simulink model "Regen_Model"  (R2023b)
settings: Solver=VariableStepAuto  StartTime=0.0  StopTime=10.0  RelTol=1e-3
undefined symbols (not defined in the file): DiscIntNeverNeededParam
settings Model: Creator=bglen  LastModifiedBy=bglen

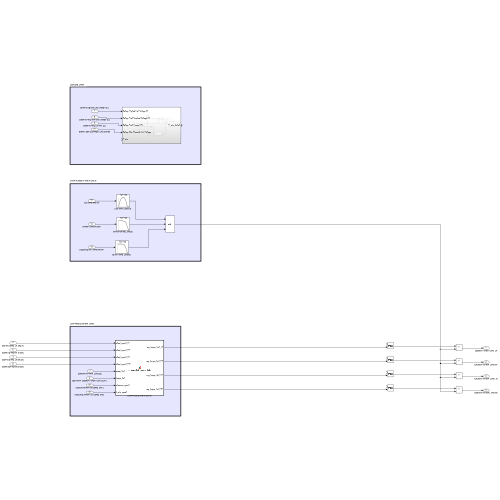
[thumbnail: Simulink's stored preview of the top-level diagram]
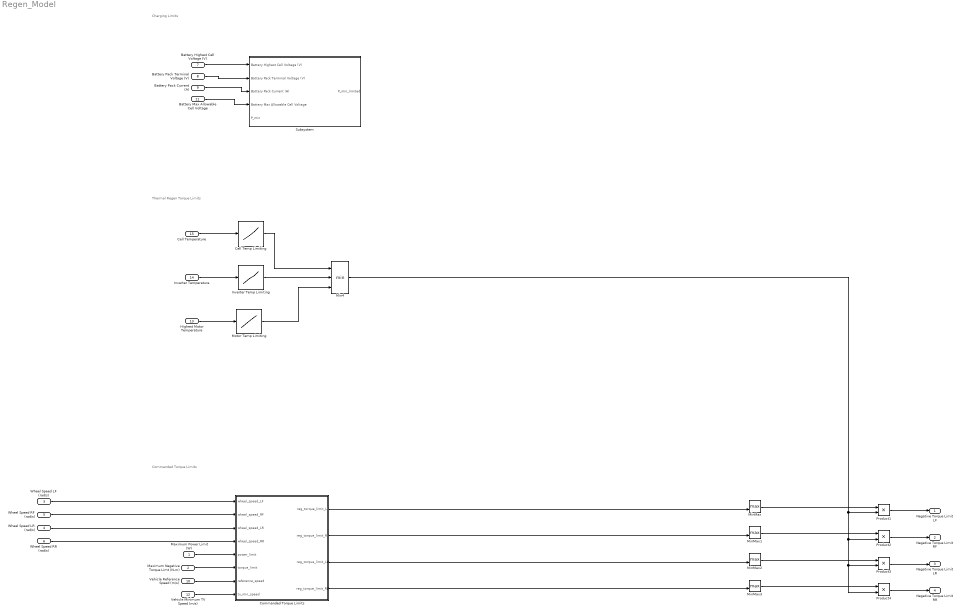
== system Regen_Model ==
  note: Commanded Torque Limits
  note: Thermal Regen Torque Limits
  note: Charging Limits
  Maximum Power Limit (W) : Inport
  Maximum Negative Torque Limt (N-m) : Inport  Port=2
  Wheel Speed LF (rad/s) : Inport  Port=3
  Wheel Speed LR (rad/s) : Inport  Port=4
  Wheel Speed RF (rad/s) : Inport  Port=5
  Wheel Speed RR (rad/s) : Inport  Port=6
  Battery Highest Cell Voltage (V) : Inport  Port=7
  Battery Pack Terminal Voltage (V) : Inport  Port=8
  Battery Pack Current (A) : Inport  Port=9
  Vehicle Reference Speed (m/s) : Inport  Port=10
  Battery Max Allowable Cell Voltage : Inport  Port=11
  Vehicle Minimum TV Speed (m/s) : Inport  Port=12
  Highest Motor Temperature : Inport  Port=13
  Inverter Temperature : Inport  Port=14
  Cell Temperature : Inport  Port=15
  Cell Temp Limiting : Lookup_n-D  NumberOfTableDimensions=1  BreakpointsForDimension1=[-15;-10;-5;0;5;10;15;20;25;30;35;40;45;50;55;60]  BreakpointsForDimension1Spacing=10  Table=[0;0.3;0.6;0.75;0.9;1;1;1;1;0.9;0.8;0.5;0.2;0.05;0;0]  InternalRulePriority=Speed  RndMeth=Simplest
  Commanded Torque Limits : MATLAB Function  TreatAsAtomicUnit=on
  Inverter Temp Limiting : Lookup_n-D  NumberOfTableDimensions=1  BreakpointsForDimension1=[0;10;20;30;40;50;60;70;80;90;100;110;120;130]  BreakpointsForDimension1Spacing=10  Table=[1;1;1;1;1;1;0.98;0.95;0.9;0.8;0.6;0.3;0.1;0]  InternalRulePriority=Speed  RndMeth=Simplest
  Min4 : MinMax  Inputs=3
  MinMax{,1..3} (4 alike) : MinMax  Function=max  Inputs=2
  Motor Temp Limiting : Lookup_n-D  NumberOfTableDimensions=1  BreakpointsForDimension1=[0;10;20;30;40;50;60;70;80;90;100;110;120;130;140]  BreakpointsForDimension1Spacing=10  Table=[1;1;1;1;1;1;1;0.98;0.95;0.9;0.8;0.6;0.3;0.1;0]  InternalRulePriority=Speed  RndMeth=Simplest
  Product{1..4} (4 alike) : Product
  Subsystem : Subsystem
  Negative Torque Limit LF : Outport
  Negative Torque Limit RF : Outport  Port=2
  Negative Torque Limit LR : Outport  Port=3
  Negative Torque Limit RR : Outport  Port=4
  wires:
  Product1/1 -> Negative Torque Limit LF/1
  Product2/1 -> Negative Torque Limit RF/1
  Product3/1 -> Negative Torque Limit LR/1
  Product4/1 -> Negative Torque Limit RR/1
  Wheel Speed LF (rad/s)/1 -> Commanded Torque Limits/1(wheel_speed_LF)
  Wheel Speed RF (rad/s)/1 -> Commanded Torque Limits/2(wheel_speed_RF)
  Wheel Speed LR (rad/s)/1 -> Commanded Torque Limits/3(wheel_speed_LR)
  Wheel Speed RR (rad/s)/1 -> Commanded Torque Limits/4(wheel_speed_RR)
  Maximum Power Limit (W)/1 -> Commanded Torque Limits/5(power_limit)
  Maximum Negative Torque Limt (N-m)/1 -> Commanded Torque Limits/6(torque_limit)
  Vehicle Minimum TV Speed (m/s)/1 -> Commanded Torque Limits/8(tv_min_speed)
  Vehicle Reference Speed (m/s)/1 -> Commanded Torque Limits/7(reference_speed)
  Highest Motor Temperature/1 -> Motor Temp Limiting/1
  Cell Temp Limiting/1 -> Min4/1
  Inverter Temp Limiting/1 -> Min4/2
  Motor Temp Limiting/1 -> Min4/3
  Cell Temperature/1 -> Cell Temp Limiting/1
  Inverter Temperature/1 -> Inverter Temp Limiting/1
  Min4/1 -> Product4/2, Product3/2, Product2/2, Product1/2
  MinMax/1 -> Product1/1
  MinMax1/1 -> Product2/1
  MinMax2/1 -> Product3/1
  MinMax3/1 -> Product4/1
  Commanded Torque Limits/4(reg_torque_limit_RR) -> MinMax3/2
  Commanded Torque Limits/3(reg_torque_limit_LR) -> MinMax2/2
  Commanded Torque Limits/2(reg_torque_limit_RF) -> MinMax1/2
  Commanded Torque Limits/1(reg_torque_limit_LF) -> MinMax/2
  Battery Highest Cell Voltage (V)/1 -> Subsystem/1(Battery Highest Cell Voltage (V))
  Battery Pack Terminal Voltage (V)/1 -> Subsystem/2(Battery Pack Terminal Voltage (V))
  Battery Pack Current (A)/1 -> Subsystem/3(Battery Pack Current (A))
  Battery Max Allowable Cell Voltage/1 -> Subsystem/4(Battery Max Allowable Cell Voltage)

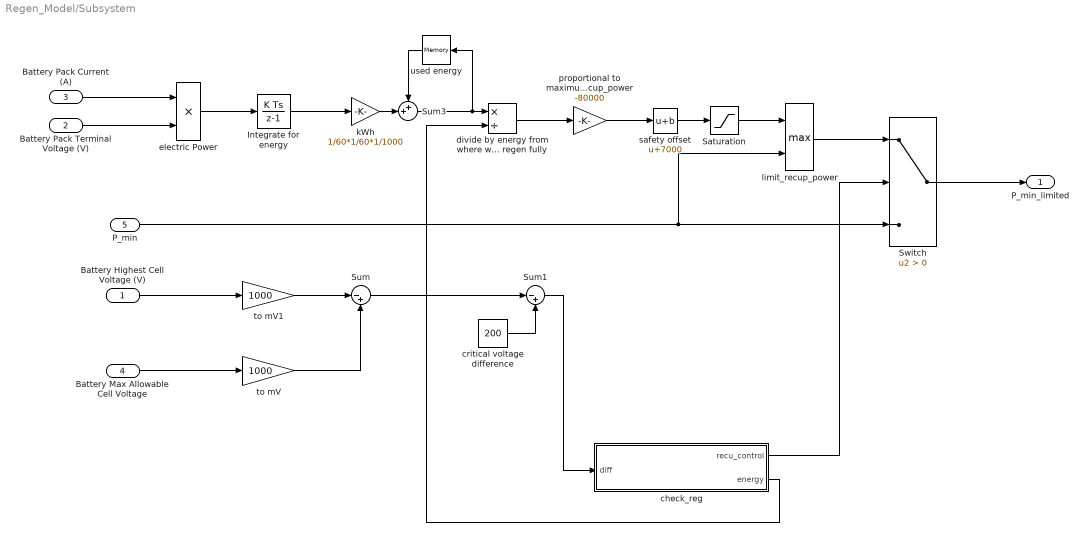
== system Regen_Model/Subsystem ==
  Battery Highest Cell Voltage (V) : Inport
  Battery Pack Terminal Voltage (V) : Inport  Port=2
  Battery Pack Current (A) : Inport  Port=3
  Battery Max Allowable Cell Voltage : Inport  Port=4
  P_min : Inport  Port=5
  Integrate for energy : DiscreteIntegrator  SampleTime=-1  ICPrevOutput=DiscIntNeverNeededParam  ICPrevScaledInput=DiscIntNeverNeededParam
  Saturation : Saturate  UpperLimit=0  LowerLimit=-100000
  Sum : Sum  Inputs=|-+
  Sum1 : Sum  Inputs=|-+
  Sum3 : Sum  Inputs=++|
  Switch : Switch  Criteria=u2 > Threshold  SaturateOnIntegerOverflow=off  InputSameDT=off
  check_reg : MATLAB Function  TreatAsAtomicUnit=on
  "critical voltage difference " : Constant  Value=200
  divide by energy from where we can use regen fully : Product  Inputs=*/
  electric Power : Product
  kWh : Gain  Gain=1/60*1/60*1/1000
  limit_recup_power : MinMax  Function=max  Inputs=2
  proportional to maximum_recup_power : Gain  Gain=-80000
  safety offset : Bias  Bias=7000  SaturateOnIntegerOverflow=off
  to mV : Gain  Gain=1000
  to mV1 : Gain  Gain=1000
  used energy : Memory  InheritSampleTime=on
  P_min_limited : Outport
  wires:
  P_min/1 -> limit_recup_power/2, Switch/3
  check_reg/2(energy) -> divide by energy from where we can use regen fully/2
  Battery Pack Current (A)/1 -> electric Power/1
  divide by energy from where we can use regen fully/1 -> proportional to maximum_recup_power/1
  limit_recup_power/1 -> Switch/1
  check_reg/1(recu_control) -> Switch/2
  used energy/1 -> Sum3/1
  to mV1/1 -> Sum/1
  proportional to maximum_recup_power/1 -> safety offset/1
  "critical voltage difference "/1 -> Sum1/2
  kWh/1 -> Sum3/2
  Sum1/1 -> check_reg/1(diff)
  Integrate for energy/1 -> kWh/1
  electric Power/1 -> Integrate for energy/1
  Sum3/1 -> divide by energy from where we can use regen fully/1, used energy/1
  safety offset/1 -> Saturation/1
  Switch/1 -> P_min_limited/1
  Sum/1 -> Sum1/1
  Saturation/1 -> limit_recup_power/1
  Battery Pack Terminal Voltage (V)/1 -> electric Power/2
  to mV/1 -> Sum/2
  Battery Max Allowable Cell Voltage/1 -> to mV/1
  Battery Highest Cell Voltage (V)/1 -> to mV1/1

== matlab function Regen_Model/Commanded Torque Limits ==
  data: wheel_speed_LF input; reg_torque_limit_LF output; reg_torque_limit_RF output; reg_torque_limit_LR output; reg_torque_limit_RR output; wheel_speed_RF input; wheel_speed_LR input; wheel_speed_RR input; power_limit input; torque_limit input; reference_speed input; tv_min_speed input
%{
Calculates regen torque limits based on wheel speeds and user set torque
limits

Note:
- regen torque is expressed as a negative
- torque_limit input is regen torque and therefore must be passed as a negative

Units:
- Power: W
- Torque: N-m
- Angular Velocity: rad/s
%}
function [reg_torque_limit_LF, reg_torque_limit_RF, reg_torque_limit_LR, reg_torque_limit_RR] = commanded_torque_limits(wheel_speed_LF, wheel_speed_RF, wheel_speed_LR, wheel_speed_RR, power_limit, torque_limit, reference_speed, tv_min_speed)

% Power (W) = Torque (N-m) * angular velocity (rad/s)
total_speed = (wheel_speed_LF + wheel_speed_RF + wheel_speed_LR + wheel_speed_RR);
total_max_torque = -(power_limit / total_speed);

% Limit based on user set max torque
if (total_max_torque < torque_limit)
    total_max_torque = torque_limit;
end

% Distribute torque limits based on a ratio of total speed
torque_limit_LF =  total_max_torque * (wheel_speed_LF / total_speed);
torque_limit_RF =  total_max_torque * (wheel_speed_RF / total_speed);
torque_limit_LR =  total_max_torque * (wheel_speed_LR / total_speed);
torque_limit_RR =  total_max_torque * (wheel_speed_RR / total_speed);

% Disable regen if below minimum speed
if (reference_speed < tv_min_speed)
    torque_limit_LF = 0;
    torque_limit_RF = 0;
    torque_limit_LR = 0;
    torque_limit_RR = 0;
end

reg_torque_limit_LF = torque_limit_LF;
reg_torque_limit_RF = torque_limit_RF;
reg_torque_limit_LR = torque_limit_LR;
reg_torque_limit_RR = torque_limit_RR;

end

== matlab function Regen_Model/Subsystem/check_reg ==
  data: diff input; recu_control output; energy output
function [recu_control, energy] = check_recu(diff)

persistent isActive

if isempty(isActive) %evaluated first time
    if diff > 0
        recu_control = 1;
        energy = diff * 0.0036 + eps;
    else
        recu_control = 0;
        energy = eps;
    end
    
    isActive.recu_contr = recu_control;
    isActive.energiemenge  = energy;

else
    recu_control = isActive.recu_contr;
    energy  = isActive.energy;
end
